simulink model "Question2"  (R2018a)
settings: Solver=VariableStepAuto  StartTime=0.0  StopTime=15  RelTol=1e-3
settings Model: Creator=e217715  LastModifiedBy=e217715

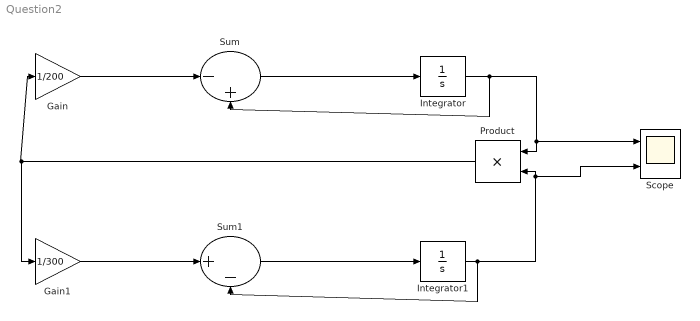
== system Question2 ==
  Gain : Gain  Gain=1/200
  Gain1 : Gain  Gain=1/300
  Integrator : Integrator  InitialCondition=400
  Integrator1 : Integrator  InitialCondition=100
  Product : Product
  Scope : Scope  NumInputPorts=2
  Sum : Sum  Inputs=|-+
  Sum1 : Sum  Inputs=|+-
  wires:
  Gain/1 -> Sum/1
  Gain1/1 -> Sum1/1
  Sum/1 -> Integrator/1
  Sum1/1 -> Integrator1/1
  Integrator/1 -> Sum/2, Product/1, Scope/1
  Integrator1/1 -> Sum1/2, Scope/2, Product/2
  Product/1 -> Gain1/1, Gain/1
